simulink model "kamman_fers"  (R2024b)
settings: Solver=VariableStepAuto  StartTime=0.0  StopTime=1000.0  RelTol=1e-3
settings Model: Creator=klyx  LastModifiedBy=klyx

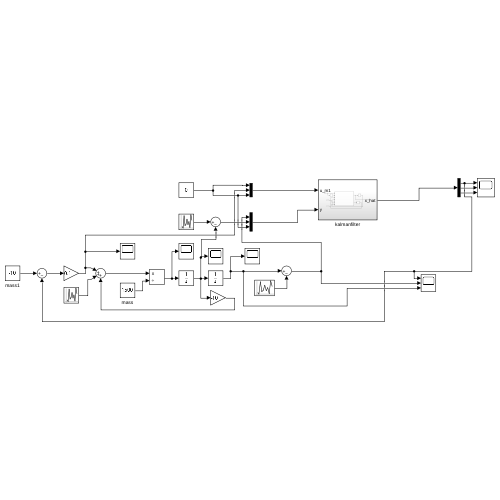
[thumbnail: Simulink's stored preview of the top-level diagram]
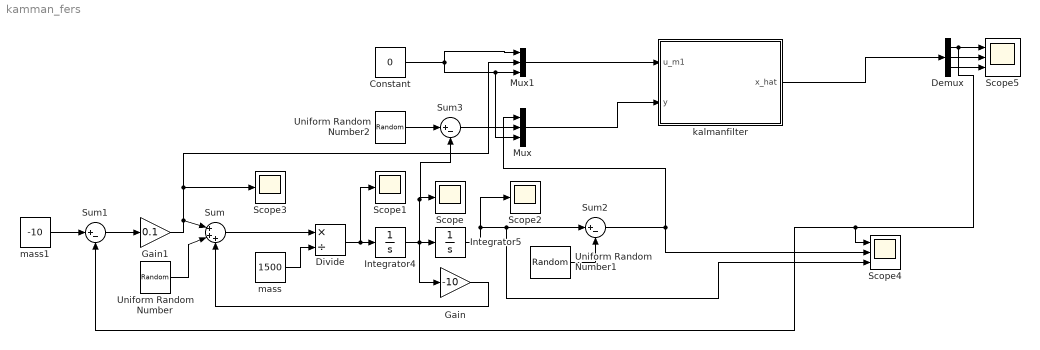
== system kamman_fers ==
  Constant : Constant  Value=0
  Demux : Demux  Outputs=3
  Divide : Product  Inputs=*/
  Gain : Gain  Gain=-10
  Gain1 : Gain  Gain=0.1
  Integrator4 : Integrator  InitialCondition=0.2
  Integrator5 : Integrator
  Mux : Mux  Inputs=3
  Mux1 : Mux  Inputs=3
  Scope{,1..3} (4 alike) : Scope
  Scope4 : Scope  NumInputPorts=3
  Scope5 : Scope  NumInputPorts=3
  Sum : Sum  Inputs=|+++
  Sum1 : Sum  Inputs=|+-
  Sum2 : Sum  Inputs=|+-
  Sum3 : Sum  Inputs=|+-
  Uniform Random Number : UniformRandomNumber  Seed=1  SampleTime=1
  Uniform Random Number1 : UniformRandomNumber  Minimum=-2  Maximum=2  Seed=1  SampleTime=1
  Uniform Random Number2 : UniformRandomNumber  Seed=1  SampleTime=1
  kalmanfilter : Subsystem
  mass : Constant  Value=1500
  mass1 : Constant  Value=-10
  wires:
  Divide/1 -> Scope1/1, Integrator4/1
  Integrator4/1 -> Sum3/2, Scope/1, Gain/1, Integrator5/1
  Sum/1 -> Divide/1
  mass/1 -> Divide/2
  Gain/1 -> Sum/3
  Integrator5/1 -> Scope4/3, Sum2/1, Scope2/1
  Gain1/1 -> Mux1/2, Scope3/1, Sum/1
  Sum1/1 -> Gain1/1
  mass1/1 -> Sum1/1
  Uniform Random Number/1 -> Sum/2
  Uniform Random Number1/1 -> Sum2/2
  Sum2/1 -> Scope4/2, Mux/1
  Constant/1 -> Mux1/1, Mux/3, Mux1/3
  Demux/1 -> Scope5/1, Sum1/2, Scope4/1
  Demux/2 -> Scope5/2
  Uniform Random Number2/1 -> Sum3/1
  Sum3/1 -> Mux/2
  Demux/3 -> Scope5/3
  Mux1/1 -> kalmanfilter/1(u_m1)
  Mux/1 -> kalmanfilter/2(y)
  kalmanfilter/1(x_hat) -> Demux/1

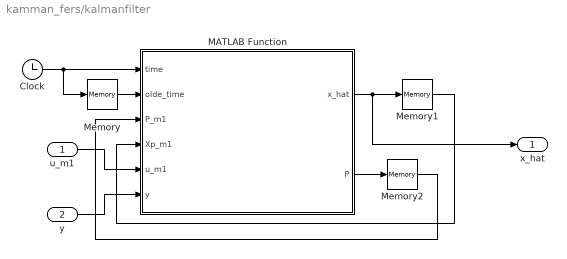
== system kamman_fers/kalmanfilter ==
  u_m1 : Inport
  y : Inport  Port=2
  Clock : Clock
  MATLAB Function : MATLAB Function  TreatAsAtomicUnit=on
  Memory : Memory
  Memory1 : Memory  InitialCondition=[0; 0.5; 0]
  Memory2 : Memory  InitialCondition=eye(3) * 1e-3
  x_hat : Outport
  wires:
  Memory/1 -> MATLAB Function/2(olde_time)
  Memory2/1 -> MATLAB Function/3(P_m1)
  MATLAB Function/2(P) -> Memory2/1
  Memory1/1 -> MATLAB Function/4(Xp_m1)
  y/1 -> MATLAB Function/6(y)
  MATLAB Function/1(x_hat) -> x_hat/1, Memory1/1
  Clock/1 -> MATLAB Function/1(time), Memory/1
  u_m1/1 -> MATLAB Function/5(u_m1)

== matlab function kamman_fers/kalmanfilter/MATLAB Function ==
  data: time input; x_hat output; olde_time input; P_m1 input; Xp_m1 input; u_m1 input; y input; P output
function [x_hat,P] = extended_kalman_filter_sim(time, olde_time, P_m1, Xp_m1, u_m1, y)
    td = time - olde_time;
    m = 1500; b = 0;
    Q_m1 = diag([1e-5, 1e-5, 1e-1]);
    %-----HS changed process noise for damping to allow faster changes ---
    %
    R =1*diag([1e-3, 1e-4, 1e-3]);
    
    h = @(xp_m1) [xp_m1(1); 0; 0];

    f = @(xp_m1, u_m1) xp_m1 + [0, 1, 0 ;0, b/m-xp_m1(3)/m, 0; 0, 0, 0]*xp_m1*td + [0,0,0;0, 1/m, 0;0,0,0]*td*u_m1;% + [0;0;Xp_m1(3)];

    F_m1 = @(xp_m1) [1, td, 0;
                     0, 1-td*xp_m1(3)/m, -td*xp_m1(2)/m;
                     0, 0, 1];

    L_m1 = @(w) [1, 0, 0;
                 0, 1, 0;
                 0, 0, 1];
    H_f = @(Xp_m1) [1, 0, 0; % C matrix
                    0, 0, 0;
                    0, 0, 0];
    
    M_f = @(Xp_m1) [1, 0, 0;
                    0, 1, 0;
                    0, 0, 1];
    H = H_f(Xp_m1);
    
    I = eye(3);
    Pm = F_m1(Xp_m1)*P_m1*F_m1(Xp_m1)'+L_m1(Xp_m1)*Q_m1*L_m1(Xp_m1)';
    Xm = f(Xp_m1,u_m1);
    
    %rank(obsv(F_m1(Xp_m1),H));
    %cond(obsv(F_m1(Xp_m1),H))

    H = H_f(Xp_m1);
    M = M_f([1;1;1]);
    K = Pm * H' / (H * Pm * H' + M * R * M');
    Xp = Xm + K*(y-h(Xp_m1));
    Pp = (I - K*H)*Pm*(I - K*H)' + K*R*K';
    P = Pp;
    x_hat = Xp;
end
